simulink model "Jang_Peter_DBIP_2017a_MinOrderObserver"  (Simulink 8.9)
settings: Solver=ode1  StartTime=0.0  StopTime=inf  FixedStep=0.002  RelTol=1e-3  EnableMultiTasking=on
values from neighbouring files (symbols this model uses):
  ALPHA_LIM_ENABLE = 1    [Jang_Peter_DBIP_setup.m]
  ALPHA_MAX = 45    [Jang_Peter_DBIP_setup.m]
  ALPHA_MIN = - ALPHA_MAX    (= -45)    [Jang_Peter_DBIP_setup.m]
  Ao = M    [Jang_Peter_DBIP_setup.m]
  Bo = [N P]    [Jang_Peter_DBIP_setup.m]
  Co = Q    [Jang_Peter_DBIP_setup.m]
  Do = [R S]    [Jang_Peter_DBIP_setup.m]
  F = [F1 F2]    [Jang_Peter_DBIP_setup.m]
  GAMMA_LIM_ENABLE = 1    [Jang_Peter_DBIP_setup.m]
  GAMMA_MAX = 25    [Jang_Peter_DBIP_setup.m]
  GAMMA_MIN = - GAMMA_MAX    (= -25)    [Jang_Peter_DBIP_setup.m]
  K_AMP = 1    [Jang_Peter_DBIP_setup.m]
  THETA_LIM_ENABLE = 1    [Jang_Peter_DBIP_setup.m]
  THETA_MAX = 90    [Jang_Peter_DBIP_setup.m]
  THETA_MIN = - THETA_MAX    (= -90)    [Jang_Peter_DBIP_setup.m]
  VMAX_DAC = 10    [Jang_Peter_DBIP_setup.m]
  wcf_1 = 2 * pi * 50.0    (= 314.159265359)    [Jang_Peter_DBIP_setup.m]
  wcf_2 = 2 * pi * 15.0    (= 94.2477796077)    [Jang_Peter_DBIP_setup.m]
  z_o = L*(C1^-1)*y_o    [Jang_Peter_DBIP_setup.m]
undefined symbols (not defined in the file or in its folder): HIL, K_ENC, qc_get_step_size, VMAX_AMP
libraries: quarc_library x10, simulink_extras x7
settings Model: Creator=MLevis  LastModifiedBy=Administrator  SimulationMode=external  ExtModeTrigDuration=15000
settings SolverCC: PositivePriorityOrder=on
settings OptimizationCC: BooleanDataType=off  OptimizeBlockIOStorage=off  BufferReuse=off  GlobalBufferReuse=off  ExpressionFolding=off  ExpressionDepthLimit=2147483647  LocalBlockOutputs=off  InitFltsAndDblsToZero=on  LifeSpan=auto
settings DebuggingCC: SaveWithParameterizedLinksMsg=none  SignalResolutionControl=TryResolveAllWithWarning  MultiTaskDSMMsg=warning  MultiTaskCondExecSysMsg=none
settings HardwareCC: ProdBitPerPointer=64  ProdBitPerSizeT=64  ProdBitPerPtrDiffT=64  ProdLargestAtomicFloat=Float  ProdIntDivRoundTo=Zero  ProdEndianess=LittleEndian  ProdWordSize=64  ProdHWDeviceType=Intel->x86-64 (Windows64)
settings ModelReferenceCC: EnableRefExpFcnMdlSchedulingChecks=off
settings RTWCC: SystemTargetFile=quarc_win64.tlc  TemplateMakefile=quarc_default_tmf  Description=QUARC Win64 Target  Toolchain=QUARC win64 | nmake (64-bit Windows)  BuildConfiguration=Faster Runs
settings STFCustomTargetCC: TargetPreCompLibLocation=C:\PROGRA~3\QUARC\lib\2017a\win64\release  ConcurrentExecutionCompliant=on  SystemTargetFile=quarc_win64.tlc
settings GRTTargetCC: TargetPreCompLibLocation=C:\PROGRA~3\QUARC\lib\2017a\win64\release  ParMdlRefBuildCompliant=off  CompOptLevelCompliant=off  GeneratePreprocessorConditionals=Use local settings  MatFileLogging=off  CPPClassGenCompliant=off  UseToolchainInfoCompliant=off  ExtMode=on  ExtModeMexFile=quarc_comm
settings ConfigComp: CovHtmlReporting=off

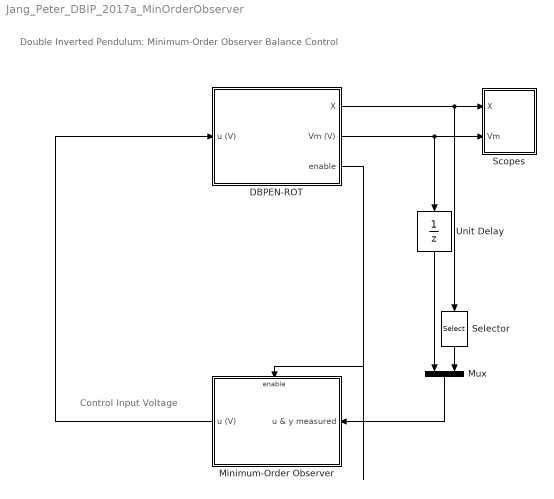
== system Jang_Peter_DBIP_2017a_MinOrderObserver ==
  note: Control Input Voltage
  note: Double Inverted Pendulum: Minimum-Order Observer Balance Control
  DBPEN-ROT : Subsystem
  Minimum-Order Observer : Subsystem  TreatAsAtomicUnit=on
  Mux : Mux  Inputs=2
  Scopes : Subsystem
  Selector : Selector  InputPortWidth=6  IndexOptions=Index vector (dialog)  Indices=[1 2 3]  OutputSizes=1
  Unit Delay : UnitDelay  SampleTime=-1
  wires:
  DBPEN-ROT/1(X) -> Scopes/1(X), Selector/1
  Minimum-Order Observer/1(u (V)) -> DBPEN-ROT/1(u (V))
  DBPEN-ROT/2(Vm (V)) -> Unit Delay/1, Scopes/2(Vm)
  DBPEN-ROT/3(enable) -> Minimum-Order Observer/Enable
  Mux/1 -> Minimum-Order Observer/1(u & y measured)
  Selector/1 -> Mux/2
  Unit Delay/1 -> Mux/1

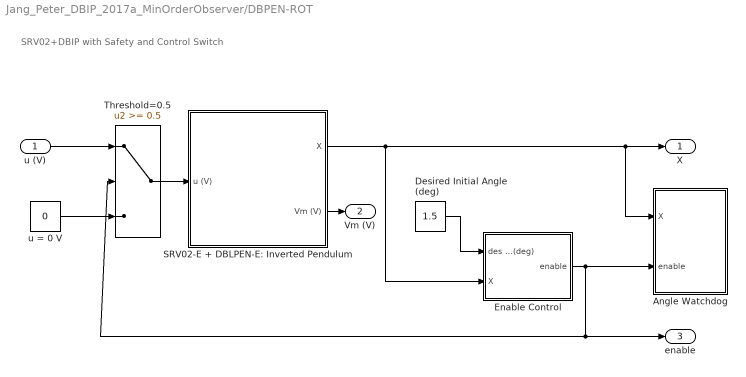
== system Jang_Peter_DBIP_2017a_MinOrderObserver/DBPEN-ROT ==
  note: SRV02+DBIP
      | with  Safety and Control Switch
  u (V) : Inport
  Angle Watchdog : Subsystem
  Desired Initial Angle (deg) : Constant  Value=1.5
  Enable Control : Subsystem
  SRV02-E + DBLPEN-E: Inverted Pendulum : Subsystem
  Threshold=0.5 : Switch  Threshold=0.5  SaturateOnIntegerOverflow=on  InputSameDT=on
  u = 0 V : Constant  Value=0
  X : Outport
  Vm (V) : Outport  Port=2
  enable : Outport  Port=3
  wires:
  SRV02-E + DBLPEN-E: Inverted Pendulum/1(X) -> Enable Control/2(X), Angle Watchdog/1(X), X/1
  Threshold=0.5/1 -> SRV02-E + DBLPEN-E: Inverted Pendulum/1(u (V))
  u (V)/1 -> Threshold=0.5/1
  u = 0 V/1 -> Threshold=0.5/3
  Desired Initial Angle (deg)/1 -> Enable Control/1(des angle (deg))
  Enable Control/1(enable) -> Angle Watchdog/2(enable), Threshold=0.5/2, enable/1
  SRV02-E + DBLPEN-E: Inverted Pendulum/2(Vm (V)) -> Vm (V)/1

== system Jang_Peter_DBIP_2017a_MinOrderObserver/Minimum-Order Observer ==
  u & y measured : Inport
  Enable : EnablePort  StatesWhenEnabling=reset
  Gain : Gain  Gain=F(1:6)  Multiplication=Matrix(K*u)
  Min-Order Observer : StateSpace  A=Ao  B=Bo  C=Co  D=Do  X0=z_o
  u (V) : Outport
  wires:
  u & y measured/1 -> Min-Order Observer/1
  Min-Order Observer/1 -> Gain/1
  Gain/1 -> u (V)/1

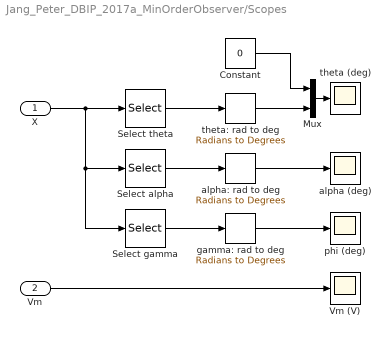
== system Jang_Peter_DBIP_2017a_MinOrderObserver/Scopes ==
  X : Inport
  Vm : Inport  Port=2
  Constant : Constant  Value=0
  Mux : Mux  Inputs=2
  Select alpha : Selector  InputPortWidth=6  IndexOptions=Index vector (dialog)  Indices=2  OutputSizes=1
  Select gamma : Selector  InputPortWidth=6  IndexOptions=Index vector (dialog)  Indices=3  OutputSizes=1
  Select theta : Selector  InputPortWidth=6  IndexOptions=Index vector (dialog)  Indices=1  OutputSizes=1
  Vm (V) : Scope
  alpha (deg) : Scope
  alpha: rad to deg : simulink_extras/Transformations/Radians to Degrees
  gamma: rad to deg : simulink_extras/Transformations/Radians to Degrees
  phi (deg) : Scope
  theta (deg) : Scope
  theta: rad to deg : simulink_extras/Transformations/Radians to Degrees
  wires:
  X/1 -> Select theta/1, Select alpha/1, Select gamma/1
  alpha: rad to deg/1 -> alpha (deg)/1
  gamma: rad to deg/1 -> phi (deg)/1
  Select theta/1 -> theta: rad to deg/1
  Select alpha/1 -> alpha: rad to deg/1
  Select gamma/1 -> gamma: rad to deg/1
  theta: rad to deg/1 -> Mux/2
  Mux/1 -> theta (deg)/1
  Vm/1 -> Vm (V)/1
  Constant/1 -> Mux/1

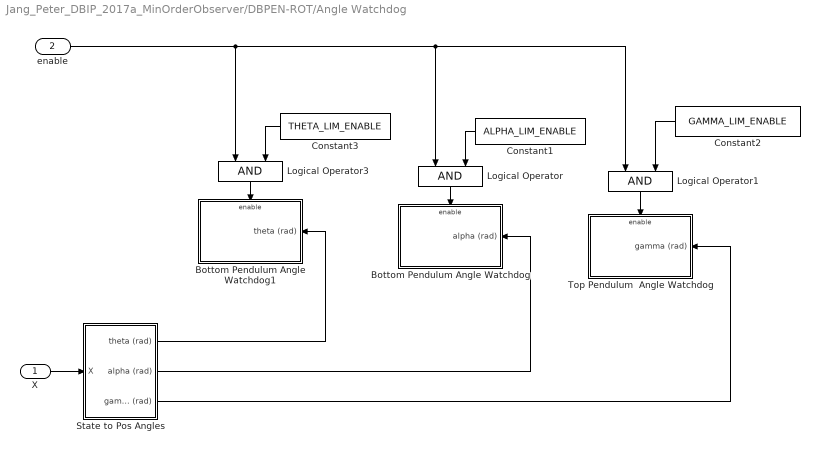
== system Jang_Peter_DBIP_2017a_MinOrderObserver/DBPEN-ROT/Angle Watchdog ==
  X : Inport
  enable : Inport  Port=2
  Bottom Pendulum Angle Watchdog : Subsystem  TreatAsAtomicUnit=on
  Bottom Pendulum Angle Watchdog1 : Subsystem  TreatAsAtomicUnit=on
  Constant1 : Constant  Value=ALPHA_LIM_ENABLE
  Constant2 : Constant  Value=GAMMA_LIM_ENABLE
  Constant3 : Constant  Value=THETA_LIM_ENABLE
  Logical Operator : Logic
  Logical Operator1 : Logic
  Logical Operator3 : Logic
  State to Pos Angles : Subsystem
  Top Pendulum  Angle Watchdog : Subsystem  TreatAsAtomicUnit=on
  wires:
  Logical Operator1/1 -> Top Pendulum  Angle Watchdog/Enable
  Constant3/1 -> Logical Operator3/2
  Logical Operator3/1 -> Bottom Pendulum Angle Watchdog1/Enable
  Constant2/1 -> Logical Operator1/2
  Constant1/1 -> Logical Operator/2
  Logical Operator/1 -> Bottom Pendulum Angle Watchdog/Enable
  X/1 -> State to Pos Angles/1(X)
  enable/1 -> Logical Operator3/1, Logical Operator/1, Logical Operator1/1
  State to Pos Angles/1(theta (rad)) -> Bottom Pendulum Angle Watchdog1/1(theta (rad))
  State to Pos Angles/2(alpha (rad)) -> Bottom Pendulum Angle Watchdog/1(alpha (rad))
  State to Pos Angles/3(gamma (rad)) -> Top Pendulum  Angle Watchdog/1(gamma (rad))

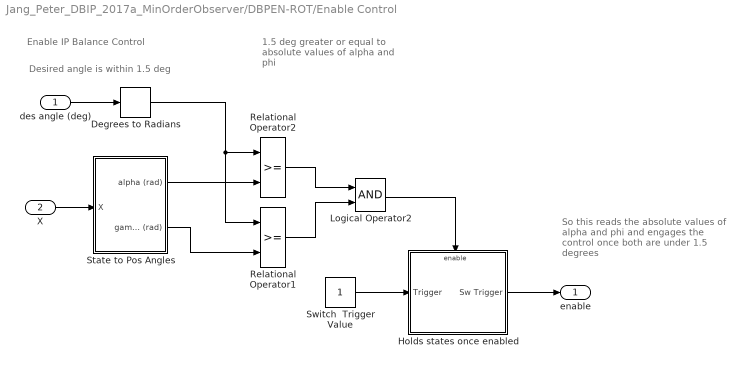
== system Jang_Peter_DBIP_2017a_MinOrderObserver/DBPEN-ROT/Enable Control ==
  note: So this reads the absolute values of alpha and phi and engages the control once both are under 1.5 degrees
  note: 1.5 deg greater or equal to absolute values of alpha and phi
  note: Desired angle is within 1.5 deg
  note: Enable IP Balance Control
  des angle (deg) : Inport
  X : Inport  Port=2
  Degrees to Radians : simulink_extras/Transformations/Degrees to Radians
  Holds states once enabled : Subsystem  TreatAsAtomicUnit=on
  Logical Operator2 : Logic
  Relational Operator1 : RelationalOperator  RndMeth=Nearest  InputSameDT=on
  Relational Operator2 : RelationalOperator  RndMeth=Nearest  InputSameDT=on
  State to Pos Angles : Subsystem
  Switch  Trigger Value : Constant
  enable : Outport
  wires:
  Relational Operator1/1 -> Logical Operator2/2
  Relational Operator2/1 -> Logical Operator2/1
  Switch  Trigger Value/1 -> Holds states once enabled/1(Trigger)
  State to Pos Angles/2(gamma (rad)) -> Relational Operator1/2
  State to Pos Angles/1(alpha (rad)) -> Relational Operator2/2
  des angle (deg)/1 -> Degrees to Radians/1
  Holds states once enabled/1(Sw Trigger) -> enable/1
  Degrees to Radians/1 -> Relational Operator2/1, Relational Operator1/1
  Logical Operator2/1 -> Holds states once enabled/Enable
  X/1 -> State to Pos Angles/1(X)

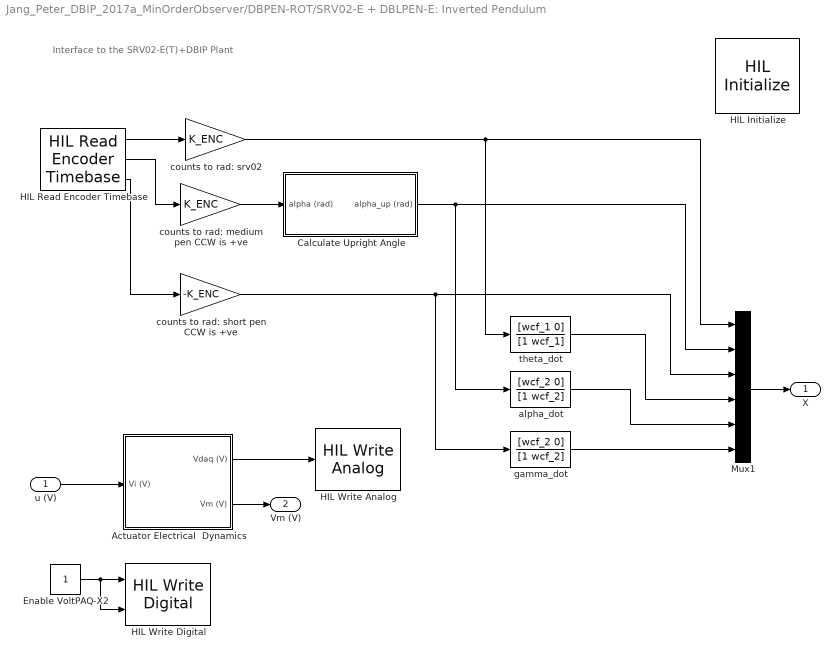
== system Jang_Peter_DBIP_2017a_MinOrderObserver/DBPEN-ROT/SRV02-E + DBLPEN-E: Inverted Pendulum ==
  note: Interface to the SRV02-E(T)+DBIP Plant
  u (V) : Inport
  Actuator Electrical  Dynamics : Subsystem
  Calculate Upright Angle : Subsystem
  Enable VoltPAQ-X2 : Constant
  HIL Initialize : quarc_library/Data Acquisition/Generic/Configuration/HIL Initialize  object_name=HIL-1  board_type=q8_usb  board_number=0  board_options=update_rate=normal  exclusive=off  active=off  hardware_clocks=[0:2]  clock_modes=[]  initial_clock_frequencies=[]  set_clock_params_at_start=off  set_clock_params_at_switch_in=off  set_clock_frequencies_at_start=off  set_clock_frequencies_at_switch_in=off  analog_input_channels=[0:7]  analog_input_configurations=[]  analog_input_maximums=10  analog_input_minimums=-10  set_analog_input_params_at_start=on  set_analog_input_params_at_switch_in=off  analog_output_channels=[0:7]  analog_output_maximums=10  analog_output_minimums=-10  initial_analog_outputs=[0]  final_analog_outputs=[0]  watchdog_analog_outputs=0  set_analog_output_params_at_start=on  set_analog_output_params_at_switch_in=off  set_analog_outputs_at_start=on  set_analog_outputs_at_switch_in=off  set_analog_outputs_at_terminate=on  set_analog_outputs_at_switch_out=off  set_analog_outputs_on_watchdog=off  digital_input_channels=[]  digital_output_channels=[0:1]  digital_output_configuration=[]  initial_digital_outputs=[0]  final_digital_outputs=[0]  watchdog_digital_outputs=[0]  set_digital_output_params_at_start=off  set_digital_output_params_at_switch_in=off  set_digital_outputs_at_start=on  set_digital_outputs_at_switch_in=off  set_digital_outputs_at_terminate=on  set_digital_outputs_at_switch_out=off  set_digital_outputs_on_watchdog=off  encoder_channels=[0:7]  quadrature=[4]  encoder_filter_frequency=[]  initial_encoder_counts=[0]  set_encoder_params_at_start=on  set_encoder_params_at_switch_in=off  set_encoder_counts_at_start=on  set_encoder_counts_at_switch_in=off  pwm_channels=[0:7]  pwm_modes=0  pwm_frequency=99.532799999999995e6/4095  pwm_configuration=[0]  pwm_alignment=[0]  pwm_polarity=[1]  pwm_leading_deadband=[0]  pwm_trailing_deadband=[0]  initial_pwm_outputs=[0]  final_pwm_outputs=[0]  watchdog_pwm_outputs=[0]  set_pwm_params_at_start=on  set_pwm_params_at_switch_in=off  set_pwm_outputs_at_start=on  set_pwm_outputs_at_switch_in=off  set_pwm_outputs_at_terminate=on  set_pwm_outputs_at_switch_out=off  set_pwm_outputs_on_watchdog=off  other_output_channels=[]  initial_other_outputs=[]  final_other_outputs=[]  watchdog_other_outputs=[]  set_other_outputs_at_start=off  set_other_outputs_at_switch_in=off  set_other_outputs_at_terminate=off  set_other_outputs_at_switch_out=off  set_other_outputs_on_watchdog=off
  HIL Read Encoder Timebase : quarc_library/Data Acquisition/Generic/Timebases/HIL Read Encoder Timebase  object_name=HIL-1  clock=0  channels=[0:2]  samples_in_buffer=max(ceil(1/qc_get_step_size), 1)  active=on  vector_output=off  data_type_mode=Inherit via back propagation  data_type=double
  HIL Write Analog : quarc_library/Data Acquisition/Generic/Immediate I//O/HIL Write Analog  object_name=HIL-1  channels=0  sample_time=-1  active=off  vector_input=off
  HIL Write Digital : quarc_library/Data Acquisition/Generic/Immediate I//O/HIL Write Digital  object_name=HIL-1  channels=[0:1]  sample_time=-1  active=off  vector_input=off
      settings: SourceProductName=QUARC Targets
  Mux1 : Mux  Inputs=6
  alpha_dot : TransferFcn  Numerator=[wcf_2 0]  Denominator=[1 wcf_2]
  counts to rad: medium pen CCW is +ve : Gain  Gain=K_ENC
  counts to rad: short pen CCW is +ve : Gain  Gain=-K_ENC
  counts to rad: srv02 : Gain  Gain=K_ENC
  gamma_dot : TransferFcn  Numerator=[wcf_2 0]  Denominator=[1 wcf_2]
  theta_dot : TransferFcn  Numerator=[wcf_1 0]  Denominator=[1 wcf_1]
  X : Outport
  Vm (V) : Outport  Port=2
  wires:
  counts to rad: srv02/1 -> Mux1/1, theta_dot/1
  theta_dot/1 -> Mux1/4
  alpha_dot/1 -> Mux1/5
  Calculate Upright Angle/1(alpha_up (rad)) -> Mux1/2, alpha_dot/1
  counts to rad: short pen CCW is +ve/1 -> Mux1/3, gamma_dot/1
  Mux1/1 -> X/1
  Actuator Electrical  Dynamics/1(Vdaq (V)) -> HIL Write Analog/1
  Enable VoltPAQ-X2/1 -> HIL Write Digital/1, HIL Write Digital/2
  HIL Read Encoder Timebase/1 -> counts to rad: srv02/1
  HIL Read Encoder Timebase/2 -> counts to rad: medium pen CCW is +ve/1
  HIL Read Encoder Timebase/3 -> counts to rad: short pen CCW is +ve/1
  counts to rad: medium pen CCW is +ve/1 -> Calculate Upright Angle/1(alpha (rad))
  u (V)/1 -> Actuator Electrical  Dynamics/1(Vi (V))
  Actuator Electrical  Dynamics/2(Vm (V)) -> Vm (V)/1
  gamma_dot/1 -> Mux1/6

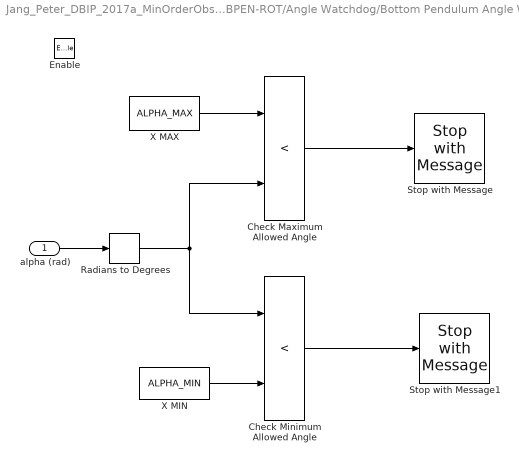
== system Jang_Peter_DBIP_2017a_MinOrderObserver/DBPEN-ROT/Angle Watchdog/Bottom Pendulum Angle Watchdog ==
  alpha (rad) : Inport
  Enable : EnablePort
  Check Maximum Allowed Angle : RelationalOperator  Operator=<  RndMeth=Nearest  InputSameDT=on
  Check Minimum Allowed Angle : RelationalOperator  Operator=<  RndMeth=Nearest  InputSameDT=on
  Radians to Degrees : simulink_extras/Transformations/Radians to Degrees
  Stop with Message : quarc_library/Sinks/Error Handling/Stop with Message  message_type=Fixed error message  message_icon=Error  message=Bottom pendulum user-defined max angle reached!
  Stop with Message1 : quarc_library/Sinks/Error Handling/Stop with Message  message_type=Fixed error message  message_icon=Error  message=Bottom pendulum user-defined min angle reached!
  X MAX : Constant  Value=ALPHA_MAX
  X MIN : Constant  Value=ALPHA_MIN
  wires:
  Radians to Degrees/1 -> Check Minimum Allowed Angle/1, Check Maximum Allowed Angle/2
  Check Maximum Allowed Angle/1 -> Stop with Message/1
  alpha (rad)/1 -> Radians to Degrees/1
  X MIN/1 -> Check Minimum Allowed Angle/2
  Check Minimum Allowed Angle/1 -> Stop with Message1/1
  X MAX/1 -> Check Maximum Allowed Angle/1

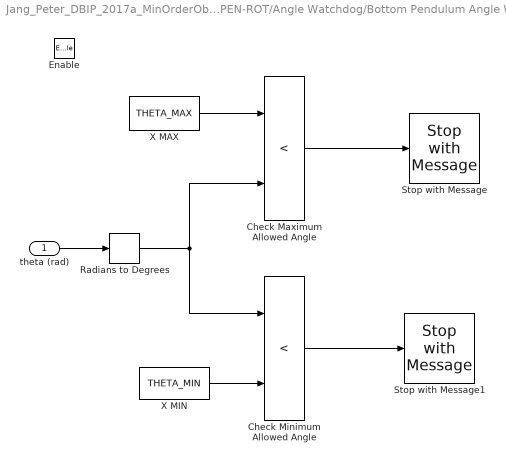
== system Jang_Peter_DBIP_2017a_MinOrderObserver/DBPEN-ROT/Angle Watchdog/Bottom Pendulum Angle Watchdog1 ==
  theta (rad) : Inport
  Enable : EnablePort
  Check Maximum Allowed Angle : RelationalOperator  Operator=<  RndMeth=Nearest  InputSameDT=on
  Check Minimum Allowed Angle : RelationalOperator  Operator=<  RndMeth=Nearest  InputSameDT=on
  Radians to Degrees : simulink_extras/Transformations/Radians to Degrees
  Stop with Message : quarc_library/Sinks/Error Handling/Stop with Message  message_type=Fixed error message  message_icon=Error  message=Rotary arm user-defined max angle reached!
  Stop with Message1 : quarc_library/Sinks/Error Handling/Stop with Message  message_type=Fixed error message  message_icon=Error  message=Rotary arm user-defined min angle reached!
  X MAX : Constant  Value=THETA_MAX
  X MIN : Constant  Value=THETA_MIN
  wires:
  X MAX/1 -> Check Maximum Allowed Angle/1
  Check Minimum Allowed Angle/1 -> Stop with Message1/1
  X MIN/1 -> Check Minimum Allowed Angle/2
  theta (rad)/1 -> Radians to Degrees/1
  Check Maximum Allowed Angle/1 -> Stop with Message/1
  Radians to Degrees/1 -> Check Maximum Allowed Angle/2, Check Minimum Allowed Angle/1

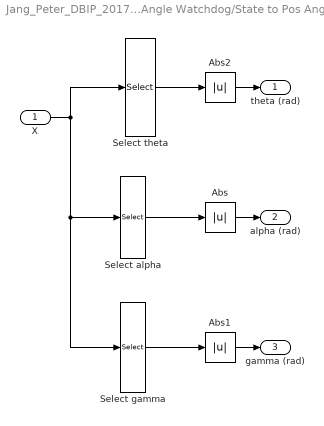
== system Jang_Peter_DBIP_2017a_MinOrderObserver/DBPEN-ROT/Angle Watchdog/State to Pos Angles ==
  X : Inport
  Abs : Abs  SaturateOnIntegerOverflow=on
  Abs1 : Abs  SaturateOnIntegerOverflow=on
  Abs2 : Abs  SaturateOnIntegerOverflow=on
  Select alpha : Selector  InputPortWidth=6  IndexOptions=Index vector (dialog)  Indices=2  OutputSizes=1
  Select gamma : Selector  InputPortWidth=6  IndexOptions=Index vector (dialog)  Indices=3  OutputSizes=1
  Select theta : Selector  InputPortWidth=6  IndexOptions=Index vector (dialog)  Indices=1  OutputSizes=1
  theta (rad) : Outport
  alpha (rad) : Outport  Port=2
  gamma (rad) : Outport  Port=3
  wires:
  Abs1/1 -> gamma (rad)/1
  Abs/1 -> alpha (rad)/1
  Abs2/1 -> theta (rad)/1
  X/1 -> Select theta/1, Select gamma/1, Select alpha/1
  Select theta/1 -> Abs2/1
  Select gamma/1 -> Abs1/1
  Select alpha/1 -> Abs/1

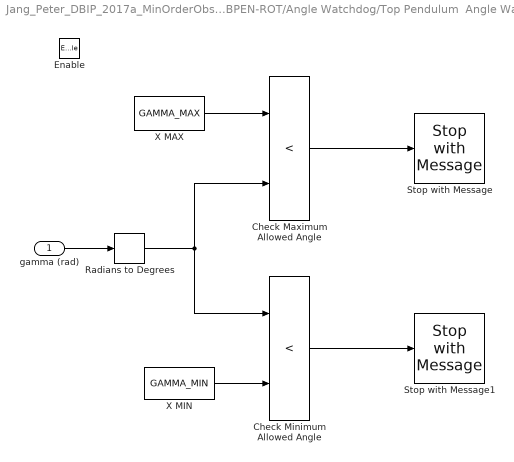
== system Jang_Peter_DBIP_2017a_MinOrderObserver/DBPEN-ROT/Angle Watchdog/Top Pendulum  Angle Watchdog ==
  gamma (rad) : Inport
  Enable : EnablePort
  Check Maximum Allowed Angle : RelationalOperator  Operator=<  RndMeth=Nearest  InputSameDT=on
  Check Minimum Allowed Angle : RelationalOperator  Operator=<  RndMeth=Nearest  InputSameDT=on
  Radians to Degrees : simulink_extras/Transformations/Radians to Degrees
  Stop with Message : quarc_library/Sinks/Error Handling/Stop with Message  message_type=Fixed error message  message_icon=Error  message=Top pendulum user-defined max angle reached!
  Stop with Message1 : quarc_library/Sinks/Error Handling/Stop with Message  message_type=Fixed error message  message_icon=Error  message=Top pendulum user-defined min angle reached!
  X MAX : Constant  Value=GAMMA_MAX
  X MIN : Constant  Value=GAMMA_MIN
  wires:
  X MAX/1 -> Check Maximum Allowed Angle/1
  Check Minimum Allowed Angle/1 -> Stop with Message1/1
  X MIN/1 -> Check Minimum Allowed Angle/2
  gamma (rad)/1 -> Radians to Degrees/1
  Check Maximum Allowed Angle/1 -> Stop with Message/1
  Radians to Degrees/1 -> Check Maximum Allowed Angle/2, Check Minimum Allowed Angle/1

== system Jang_Peter_DBIP_2017a_MinOrderObserver/DBPEN-ROT/Enable Control/Holds states once enabled ==
  Trigger : Inport
  Enable : EnablePort
  Sw Trigger : Outport  InitialOutput=[0]
  wires:
  Trigger/1 -> Sw Trigger/1

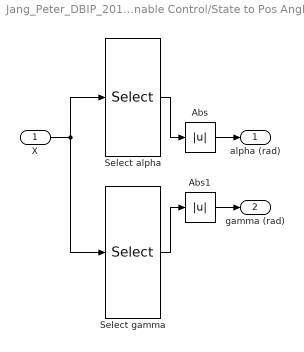
== system Jang_Peter_DBIP_2017a_MinOrderObserver/DBPEN-ROT/Enable Control/State to Pos Angles ==
  X : Inport
  Abs : Abs  SaturateOnIntegerOverflow=on
  Abs1 : Abs  SaturateOnIntegerOverflow=on
  Select alpha : Selector  InputPortWidth=6  IndexOptions=Index vector (dialog)  Indices=2  OutputSizes=1
  Select gamma : Selector  InputPortWidth=6  IndexOptions=Index vector (dialog)  Indices=3  OutputSizes=1
  alpha (rad) : Outport
  gamma (rad) : Outport  Port=2
  wires:
  Select alpha/1 -> Abs/1
  Select gamma/1 -> Abs1/1
  X/1 -> Select alpha/1, Select gamma/1
  Abs/1 -> alpha (rad)/1
  Abs1/1 -> gamma (rad)/1

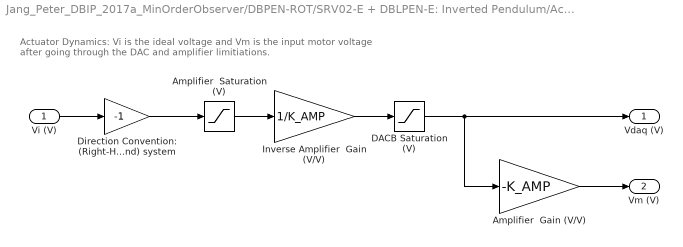
== system Jang_Peter_DBIP_2017a_MinOrderObserver/DBPEN-ROT/SRV02-E + DBLPEN-E: Inverted Pendulum/Actuator Electrical  Dynamics ==
  note: Actuator Dynamics: Vi is the ideal voltage and Vm is the
      | input motor voltage after going through the DAC and amplifier limitiations.
  Vi (V) : Inport
  Amplifier  Gain (V/V) : Gain  Gain=-K_AMP
  Amplifier  Saturation (V) : Saturate  UpperLimit=VMAX_AMP  LowerLimit=-VMAX_AMP
  DACB Saturation (V) : Saturate  UpperLimit=VMAX_DAC  LowerLimit=-VMAX_DAC
  Direction Convention: (Right-Hand) system : Gain  Gain=-1  SaturateOnIntegerOverflow=on  OutDataTypeStr=Inherit: Same as input  ParamDataTypeStr=Inherit: Same as input
  Inverse Amplifier  Gain (V/V) : Gain  Gain=1/K_AMP
  Vdaq (V) : Outport
  Vm (V) : Outport  Port=2
  wires:
  Vi (V)/1 -> Direction Convention: (Right-Hand) system/1
  Amplifier  Saturation (V)/1 -> Inverse Amplifier  Gain (V/V)/1
  Inverse Amplifier  Gain (V/V)/1 -> DACB Saturation (V)/1
  DACB Saturation (V)/1 -> Amplifier  Gain (V/V)/1, Vdaq (V)/1
  Amplifier  Gain (V/V)/1 -> Vm (V)/1
  Direction Convention: (Right-Hand) system/1 -> Amplifier  Saturation (V)/1

== system Jang_Peter_DBIP_2017a_MinOrderObserver/DBPEN-ROT/SRV02-E + DBLPEN-E: Inverted Pendulum/Calculate Upright Angle ==
  alpha (rad) : Inport
  Math Function : Math  Operator=mod  SaturateOnIntegerOverflow=on
  Mod Angle  (rad) : Constant  Value=2*pi
  Offset Angle  (rad) : Constant  Value=-pi
  Sum : Sum  SaturateOnIntegerOverflow=on  InputSameDT=on  OutDataTypeStr=Inherit: Same as first input
  alpha_up (rad) : Outport
  wires:
  Sum/1 -> alpha_up (rad)/1
  Mod Angle  (rad)/1 -> Math Function/2
  Offset Angle  (rad)/1 -> Sum/2
  alpha (rad)/1 -> Math Function/1
  Math Function/1 -> Sum/1
